simulink model "templateVFreplay"  (R2019b)
settings: Solver=ode23tb  StartTime=0  StopTime=dataSim(l).Time(end)  FixedStep=Ts
model workspace (MAT data in the model file):
  AC8B_test_sdosession : sldodialogs.data.SessionData (value not decoded)
  tp34291882_bceb_4da8_b486_81ba615ab517 = [0 0.0333333 0.0666667 0.1 0.1333334 0.1666667 0.2 0.2333333 0.2666666 0.2999999 0.3333332 0.3666665 ... (13500 elements, 2700x5)]
  tp5fd81924_c6b2_4820_a4c1_c746ac51258e : object (value not decoded)
  tp61e2f470_2812_498a_af75_e87b8b944307 = [0 0.0333333 0.0666667 0.1 0.1333334 0.1666667 0.2 0.2333333 0.2666666 0.2999999 0.3333332 0.3666665 ... (13500 elements, 2700x5)]
  tpfa3056f0_c430_45b3_969f_b76cef1498ad : object (value not decoded)
undefined symbols (not defined in the file): dataSim, dyn, Fnom, g, gcbh, genTpd0, genTppd0, genTppq0, genTpq0, genXd, genXl, genXpd, genXppd, genXppq, genXpq, genXq, govDisable, ifd, init, j, l, MBase, p, sps_rtmsupport, sys, Tb1, Tc1, Vnom, vt
libraries: powerlib x28, modelLibrary x22, simulink x15, powerlib_meascontrol x5, spsST2AModel x4, GenLib x2, ideal_source x1
(part 2 of 4)

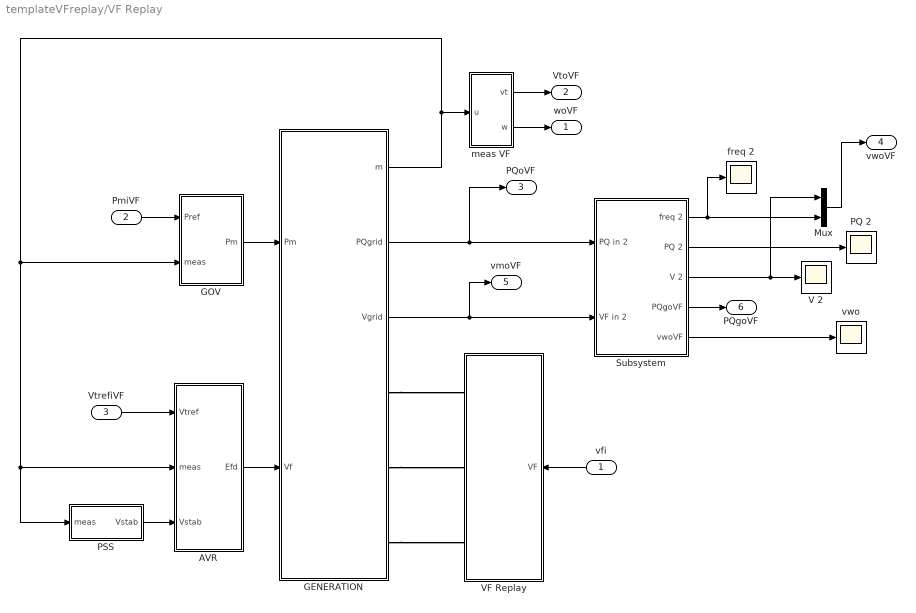
== system templateVFreplay/VF Replay ==
  vfi : Inport  PortDimensions=2
  PmiVF : Inport  Port=2
  VtrefiVF : Inport  Port=3
  AVR : Subsystem  BlockChoice=ST4B  VariantControlMode=Label  Variant=on  LabelModeActiveChoice=Variant1
      settings: AttributesFormatString=%<BlockChoice>
  GENERATION : Subsystem  VariantControlMode=Label  Variant=on  LabelModeActiveChoice=Variant2
      settings: AttributesFormatString=%<BlockChoice>
  GOV : Subsystem  BlockChoice=GGOV1  VariantControlMode=Label  Variant=on  LabelModeActiveChoice=Variant1
      settings: AttributesFormatString=%<BlockChoice>
  Mux : Mux  Inputs=2
  PQ 2 : Scope
  PSS : Subsystem  BlockChoice=PSS2B  VariantControlMode=Label  Variant=on  VariantControl=on  LabelModeActiveChoice=Variant2
      settings: AttributesFormatString=%<BlockChoice>
  Subsystem : Subsystem
  V 2 : Scope
  VF Replay : Subsystem
  freq 2 : Scope
  meas VF : Subsystem
  vwo : Scope
  woVF : Outport  VectorParamsAs1DForOutWhenUnconnected=off
  VtoVF : Outport  Port=2  VectorParamsAs1DForOutWhenUnconnected=off
  PQoVF : Outport  Port=3  SampleTime=1/30  VectorParamsAs1DForOutWhenUnconnected=off
  vwoVF : Outport  Port=4  VectorParamsAs1DForOutWhenUnconnected=off
  vmoVF : Outport  Port=5  VectorParamsAs1DForOutWhenUnconnected=off
  PQgoVF : Outport  Port=6  SampleTime=1/30  VectorParamsAs1DForOutWhenUnconnected=off
  wires:
  GENERATION/3(Vgrid) -> vmoVF/1, Subsystem/2(VF in 2)
  GENERATION/1(m) -> PSS/1(meas), AVR/2(meas), GOV/2(meas), meas VF/1(u)
  GENERATION/2(PQgrid) -> PQoVF/1, Subsystem/1(PQ in 2)
  vfi/1 -> VF Replay/1(VF)
  meas VF/1(vt) -> VtoVF/1
  meas VF/2(w) -> woVF/1
  Subsystem/1(freq 2) -> Mux/2, freq 2/1
  Subsystem/2(PQ 2) -> PQ 2/1
  Subsystem/4(PQgoVF) -> PQgoVF/1
  Subsystem/3(V 2) -> V 2/1, Mux/1
  Subsystem/5(vwoVF) -> vwo/1
  Mux/1 -> vwoVF/1
  VtrefiVF/1 -> AVR/1(Vtref)
  PmiVF/1 -> GOV/1(Pref)
  GOV/1(Pm) -> GENERATION/1(Pm)
  PSS/1(Vstab) -> AVR/3(Vstab)
  AVR/1(Efd) -> GENERATION/2(Vf)
  connections:
  GENERATION/RConn1 -- VF Replay/RConn1
  GENERATION/RConn2 -- VF Replay/RConn2
  GENERATION/RConn3 -- VF Replay/RConn3

== system templateVFreplay/view ==
  Gain : Gain  Gain=1/MBase
  Selector2 : Selector  InputPortWidth=4  IndexOptions=Index vector (dialog)  Indices=[2 4]  OutputSizes=1
  Selector3 : Selector  InputPortWidth=4  IndexOptions=Index vector (dialog)  Indices=[1 3]  OutputSizes=1
  P : Outport  VectorParamsAs1DForOutWhenUnconnected=off
  Q : Outport  Port=2  VectorParamsAs1DForOutWhenUnconnected=off
  wires:
  [PQ_2] -> Gain/1
  Gain/1 -> Selector2/1, Selector3/1
  Selector2/1 -> Q/1
  Selector3/1 -> P/1

== system templateVFreplay/VF Replay/AVR ==
  Vtref : Inport
  meas : Inport  Port=2
  Vstab : Inport  Port=3
  REXS : Subsystem  VariantControl=Variant1  mask{p=dyn.rexs_102_GAS}
      mask prompts: p "Parameters"
      mask DialogControl DescGroupVar Prompt: REXS
  ST1A : Subsystem  VariantControl=Variant2  mask{p=dyn.esst1a_102_HYDRO}
      mask prompts: p "Parameters"
      mask DialogControl DescGroupVar Prompt: ST1A
  ST4B : Subsystem  VariantControl=Variant3  mask{p=dyn.esst4b_102_STEAM}
      mask prompts: p "Parameters"
      mask DialogControl DescGroupVar Prompt: ST4B
  Efd : Outport  VectorParamsAs1DForOutWhenUnconnected=off

== system templateVFreplay/VF Replay/GENERATION ==
  Pm : Inport
  Vf : Inport  Port=2
  GENROU_TERMINAL : Subsystem  VariantControl=Variant1  mask{g=sys.GENERATOR(1), p=dyn.genrou_31923_COLUSGT1}
      mask prompts: g "Generator Parameters"; p "Dynamic Parameters"
      mask DialogControl DescGroupVar Prompt: GENROU_TRANSFORMER
  GENROU_TRANSFORMER : Subsystem  VariantControl=Variant2  mask{g=sys.GENERATOR(2), t=sys.TRANSFORMER, p=dyn.genrou_102_GAS}
      mask prompts: g "Generator Parameters"; t "Transformer Parameters"; p "Dynamic Parameters"
      mask DialogControl DescGroupVar Prompt: GENROU_TRANSFORMER
  GENSAL_TRANSFORMER : Subsystem  VariantControl=Variant3  mask{g=sys.GENERATOR(2), t=sys.TRANSFORMER, p=dyn.gentpj_102_HYDRO}
      mask prompts: g "Generator Parameters"; t "Transformer Parameters"; p "Dynamic Parameters"
      mask DialogControl DescGroupVar Prompt: GENSAL_TRANSFORMER
  GENTPJ_TERMINAL : Subsystem  VariantControl=Variant4  mask{g=g, t=t, p=p}
      mask prompts: g "Generator Parameters"; t "Transformer Parameters"; p "Dynamic Parameters"
      mask DialogControl DescGroupVar Prompt: GENTPJ_TRANSFORMER
  GENTPJ_TRANSFORMER : Subsystem  VariantControl=Variant5  mask{g=sys.GENERATOR(2), t=sys.TRANSFORMER, p=dyn.genrou_102_GAS}
      mask prompts: g "Generator Parameters"; t "Transformer Parameters"; p "Dynamic Parameters"
      mask DialogControl DescGroupVar Prompt: GENTPJ_TRANSFORMER
  A : PMIOPort  Side=Right
  B : PMIOPort  Port=2  Side=Right
  C : PMIOPort  Port=3  Side=Right
  m : Outport  VectorParamsAs1DForOutWhenUnconnected=off
  PQgrid : Outport  Port=2  VectorParamsAs1DForOutWhenUnconnected=off
  Vgrid : Outport  Port=3  VectorParamsAs1DForOutWhenUnconnected=off

== system templateVFreplay/VF Replay/GOV ==
  Pref : Inport
  meas : Inport  Port=2
  GGOV1 : Subsystem  VariantControl=Variant1  mask{p=dyn.ggov1_102_GAS, g=sys.GENERATOR(2)}
      mask prompts: p "Parameters"; g "generator"
      mask DialogControl DescGroupVar Prompt: GGOV1
  IEEEG3 : Subsystem  VariantControl=Variant2  mask{p=dyn.ieeeg3_102_HYDRO}
      mask prompts: p "Parameters"
      mask DialogControl DescGroupVar Prompt: IEEEG3
  Pm : Outport  VectorParamsAs1DForOutWhenUnconnected=off

== system templateVFreplay/VF Replay/PSS ==
  meas : Inport
  PSS1A : Subsystem  VariantControl=Variant1  mask{p=dyn.pss1a_102_HYDRO}
      mask prompts: p "Parameters"
      mask DialogControl DescGroupVar Prompt: PSS1A
  PSS2A : Subsystem  VariantControl=Variant2  mask{p=dyn.pss2a_102_GAS}
      mask prompts: p "Parameters"
      mask DialogControl DescGroupVar Prompt: PSS2A
  PSS2B : Subsystem  VariantControl=Variant3  mask{p=dyn.pss2b_102_STEAM}
      mask prompts: p "Parameters"
      mask DialogControl DescGroupVar Prompt: PSS2B
  Vstab : Outport  VectorParamsAs1DForOutWhenUnconnected=off

== system templateVFreplay/VF Replay/Subsystem ==
  PQ in 2 : Inport
  VF in 2 : Inport  Port=2
  PQ VF : Subsystem
  PQ VF comp : Subsystem
  V VF comp : Subsystem
  VF VF : Subsystem
  freq : Subsystem
  freq 2 : Outport  VectorParamsAs1DForOutWhenUnconnected=off
  PQ 2 : Outport  Port=2  VectorParamsAs1DForOutWhenUnconnected=off
  V 2 : Outport  Port=3  VectorParamsAs1DForOutWhenUnconnected=off
  PQgoVF : Outport  Port=4  VectorParamsAs1DForOutWhenUnconnected=off
  vwoVF : Outport  Port=5  VectorParamsAs1DForOutWhenUnconnected=off
  tag scope: PQ_2=global, PQoVF=global
  wires:
  V VF comp/1(y) -> V 2/1
  VF in 2/1 -> V VF comp/1(u), VF VF/1(u)
  PQ VF comp/1("y ") -> [PQ_2], PQ 2/1
  freq/1(y) -> freq 2/1
  PQ VF/1(y) -> PQgoVF/1
  VF VF/1(y) -> vwoVF/1
  PQ in 2/1 -> [PQoVF], PQ VF/1(u), PQ VF comp/1(u)

== system templateVFreplay/VF Replay/VF Replay ==
  VF : Inport
  Constant1 : Constant
  Demux : Demux  Outputs=2
  Gain : Gain  Gain=2*pi*60
  Gain7 : Gain  Gain=1e3*sqrt(2/3)
  Gain8 : Gain  Gain=2*pi*60
  Ideal Source (custom) : ideal_source/Ideal Source (custom)  InternalConnection=Yg  VoltagePhases=off  Voltage=sys.BUS(1).VBUS*1e3  PhaseAngle=0  Voltage_phases=[25e3 25e3 25e3]/sqrt(3)  PhaseAngles_phases=[0 -120 +120]  Frequency=60  NonIdealSource=on  SpecifyImpedance=off  Resistance=1e-5  Inductance=1e-5  ShortCircuitLevel=100e6  BaseVoltage=sys.BUS(1).VBUS*1e3  XRratio=7  BusType=swing  Pref=10e3  Qref=0  Prefabc=[10e3, 10e3, 10e3]  Qrefabc=[0, 0, 0]  Qmin=-inf  Qmax=inf
  Sum : Sum  Inputs=|+-
  theta integrator : Integrator  InitialCondition=2*pi*60
  theta integrator1 : Integrator  InitialCondition=2*pi*60
  A : PMIOPort  Side=Right
  B : PMIOPort  Port=2  Side=Right
  C : PMIOPort  Port=3  Side=Right
  wires:
  theta integrator/1 -> Sum/1
  Constant1/1 -> Gain8/1
  Gain7/1 -> Ideal Source (custom)/2
  VF/1 -> Demux/1
  Demux/2 -> Gain/1
  Gain/1 -> theta integrator/1
  Sum/1 -> Ideal Source (custom)/1
  Demux/1 -> Gain7/1
  theta integrator1/1 -> Sum/2
  Gain8/1 -> theta integrator1/1
  connections:
  Ideal Source (custom)/RConn2 -- B/RConn1
  Ideal Source (custom)/RConn1 -- C/RConn1
  Ideal Source (custom)/RConn3 -- A/RConn1

== system templateVFreplay/VF Replay/meas VF ==
  u : Inport
  Bus Selector6 : BusSelector  OutputSignals="dq0 components.Stator voltage  vd (pu),dq0 components.Stator voltage  vq (pu),Mechanical.Rotor speed  wm  (pu)"
  Euclidian Norm5 : Subsystem
  wo VF : Subsystem
  vt : Outport  VectorParamsAs1DForOutWhenUnconnected=off
  w : Outport  Port=2  VectorParamsAs1DForOutWhenUnconnected=off
  wires:
  u/1 -> Bus Selector6/1
  Bus Selector6/2 -> Euclidian Norm5/2(u2)  "<Stator voltage  vq (pu)>"
  Bus Selector6/1 -> Euclidian Norm5/1(u1)  "<Stator voltage  vd (pu)>"
  Euclidian Norm5/1(y) -> vt/1  "vt"
  Bus Selector6/3 -> wo VF/1(u)  "<Rotor speed  wm  (pu)>"
  wo VF/1(y) -> w/1

== system templateVFreplay/VF Replay/AVR/REXS ==
  Vtref : Inport
  meas : Inport  Port=2
  Vstab : Inport  Port=3
  Bus Selector1 : BusSelector  OutputSignals="dq0 components.Stator voltage  vd (pu),dq0 components.Stator voltage  vq (pu),dq0 components.Stator current  id (pu),dq0 components.Stator current  iq (pu),dq0 components.Field current  ifd (pu)"
  Euclidian Norm3 : Subsystem
  Euclidian Norm4 : Subsystem
  "Rotating Excitation System (Continuous) " : Subsystem  mask(PSS1A - Single Input Power System Stabilizer){Tr=p.tr, Kvp=p.kvp, Kvi=p.kvi, Vimax=p.vimax, Ta=p.ta, Tb=[p.tb1 p.tb2], Tc=[p.tc1 p.tc2], Vrrange=[p.vrmin p.vrmax], Kf=p.kf, Tf=p.tf, Tfll=[p.tf1 p.tf2], Fbf=p.fbf, Kip=p.kip, Kii=p.kii, Tp=p.tp, Kh=p.kh, Ke=p.ke, Te=p.te, Vfrange=[p.vfmin p.vfmax], Kc=p.kc, Kd=p.kd, E=[p.e1 p.e2], Se=[p.se1 p.se2], Xc=p.xc, Vcmax=p.vcmax, Kefd=p.kefd}
      mask prompts: Tr "Tr, Voltage Transducer Time Constant [s]"; Kvp "Kvp, Proportional Gain"; Kvi "Kvi, Integral Gain"; Vimax "Vimax, Input Limit [pu]"; Ta "Ta, Time Constant [s]"; Tb "Tb, Lag Time Constants [s]"; Tc "Tc, Lead Time Constants [s]"; Vrrange "[Vrmin Vrmax], Output Range [pu]"; Kf "Kf, Rate Gain"; Tf "Tf, Rate Time Constant [s]"; Tfll "[Tf1 Tf2], Lead/lag Contants [s]"; Fbf "Fbf, Feedback Signal Fl"; Kip "Kip, Regulator Proportional Gain"; Kii "Kii, Regulator Inegral Gain"; Tp "Tp, Bridge Time Constant [s]"; Kh "Kh, Voltage Controller Gain"; Ke "Ke, Exciter Proportional Constant"; Te "Te, Exciter Time Constant [s]"; Vfrange "[Vfmin Vfmax], Field Current Bounds [pu]"; Kc "Kc, Rectifier Regulation Factor [pu]"; Kd "Kd, Exciter Regulation Factor [pu]"; E "[E1 E2], Field Voltage Value Saturation"; Se "[Se1 Se2], Saturation Factor"; Xc "Xc,  Compounding Reactance [pu]"; Vcmax "Vcmax, Maximum Compounding Voltage [pu]"; Kefd "Kefd, Field Voltage Feedback"
      mask init:
      | % Extract Parameters
      | Tb1 = Tb(1);        Tb2 = Tb(2);
      | Tc1 = Tc(1);        Tc2 = Tc(2);
      | Tf1 = Tfll(1);      Tf2 = Tfll(2);
      | Vrmin = Vrrange(1); Vrmax = Vrrange(2);
      | Vfmin = Vfrange(1); Vfmax = Vfrange(2);
      mask DialogControl Container9 Prompt: Voltage Regulator
      mask DialogControl Container11 Prompt: Feedback Dynamics
      mask DialogControl Container25 Prompt: Field Current Regulator
      mask DialogControl Container29 Prompt: Rotating Exciter
      mask Display:
      | port_label('input',1,'Vref');
      | port_label('input',2,'Vt');
      | port_label('input',3,'It');
      | port_label('input',4,'Ifd');
      | port_label('input',5,'Vstab');
      | port_label('output',1,'Efd');
      | 
      | color('blue');disp('AVR/Exciter')
  Efd : Outport  VectorParamsAs1DForOutWhenUnconnected=off
  wires:
  Vstab/1 -> "Rotating Excitation System (Continuous) "/5(Vstab)
  Bus Selector1/1 -> Euclidian Norm3/1(u1)  "<Stator voltage  vd (pu)>"
  Vtref/1 -> "Rotating Excitation System (Continuous) "/1(Vref)
  Bus Selector1/3 -> Euclidian Norm4/1(u1)  "<Stator current  id (pu)>"
  Euclidian Norm4/1(y) -> "Rotating Excitation System (Continuous) "/3(It)  "It"
  Bus Selector1/4 -> Euclidian Norm4/2(u2)  "<Stator current  iq (pu)>"
  Bus Selector1/2 -> Euclidian Norm3/2(u2)  "<Stator voltage  vq (pu)>"
  Euclidian Norm3/1(y) -> "Rotating Excitation System (Continuous) "/2(Vt)  "Vt"
  Bus Selector1/5 -> "Rotating Excitation System (Continuous) "/4(Ifd)  "<Field current  ifd (pu)>"
  "Rotating Excitation System (Continuous) "/1(Efd) -> Efd/1
  meas/1 -> Bus Selector1/1

== system templateVFreplay/VF Replay/AVR/ST1A ==
  Vtref : Inport
  meas : Inport  Port=2
  Vstab : Inport  Port=3
  Bus Selector8 : BusSelector  OutputSignals="dq0 components.Field current  ifd (pu),dq0 components.Stator voltage  vd (pu),dq0 components.Stator voltage  vq (pu),dq0 components.Stator current  id (pu),dq0 components.Stator current  iq (pu)"
  Euclidian Norm1 : Subsystem
  Mux1 : Mux  Inputs=2
  Mux4 : Mux  Inputs=2
  ST1A Excitation System : Subsystem  DialogController=POWERSYS.PowerSysDialog  LoadFcn=sps_rtmsupport('LoadFcn', gcbh);  StartFcn=sps_rtmsupport('StartFcn', gcbh);  StopFcn=sps_rtmsupport('StopFcn', gcbh);  mask(ST1A Excitation System){Tr=20e-3, KaTa=[p.ka p.ta], VIminmax=[p.vimin p.vimax], VAminmax=[p.vamin p.vamax], VRminmax=[p.vrmin p.vrmax], KfTf=[p.kf p.tf], TbTc=[p.tb p.tc p.tb1 p.tc1], KLR=p.klr, ILR=p.ilr, Kc=p.kc, v0=[1 1], TsBlock=0}
      mask prompts: Tr "Low-pass filter time constant Tr(s):"; KaTa "Voltage regulator gain and time constant [Ka Ta(s)]:"; VIminmax "Voltage regulator input limits [VImin(pu) VImax(pu)]:"; VAminmax "Voltage regulator internal limits [VAmin(pu) VAmax(pu)]:"; VRminmax "Voltage regulator output limits [VRmin(pu) VRmax(pu)]:"; KfTf "Damping filter gain and time constant [Kf Tf(s)]:"; TbTc "Transient gain reduction lead and lag time constants [Tb(s) Tc(s) Tb1(s) Tc1(s)]:"; KLR "Exciter output current limiter gain KLR(pu):"; ILR "Exciter output current limit reference ILR(pu):"; Kc "Rectifier loading factor Kc(pu):"; v0 "Initial values of terminal voltage and field voltage [Vt0(pu) Efd0(pu)]:"; TsBlock "Sample time:"
      mask help: Implements a synchronous machine voltage regulator and exciter based on the IEEE type ST1A excitation system model. The output is the field voltage to apply to the Vf input of a Synchronous Machine block. Inputs and output are in p.u.
      mask init:
      | Ka = KaTa(1);
      | Ta = KaTa(2);
      | 
      | Kf = KfTf(1);
      | Tf = KfTf(2);
      | 
      | Tb = TbTc(1);
      | Tc = TbTc(2);
      settings: CopyFcn=sps_rtmsupport('CopyFcn', gcbh);  DeleteFcn=sps_rtmsupport('DeleteFcn', gcbh);  UndoDeleteFcn=sps_rtmsupport('UndoDeleteFcn', gcbh);  ModelCloseFcn=sps_rtmsupport('ModelCloseFcn', gcbh);  PreSaveFcn=sps_rtmsupport('PreSaveFcn', gcbh);  PostSaveFcn=sps_rtmsupport('PostSaveFcn', gcbh);  NameChangeFcn=sps_rtmsupport('NameChangeFcn', gcbh);  PreCopyFcn=sps_rtmsupport('PreCopyFcn', gcbh);  OpenFcn=sps_rtmsupport('OpenFcn', gcbh, []);  CloseFcn=sps_rtmsupport('CloseFcn', gcbh);  PreDeleteFcn=sps_rtmsupport('PreDeleteFcn', gcbh);
      mask Help: helpview(psbhelp);
      mask DialogControl ParameterTabVar0 Prompt: Controllers
      mask DialogControl ParameterTabVar01 Prompt: Exciter and Rectifier
      mask DialogControl ParameterTabVar012 Prompt: Initial Values
      mask Display: color('blue');disp('ST1A')
  Terminator : Terminator
  Efd : Outport  VectorParamsAs1DForOutWhenUnconnected=off
  wires:
  Mux1/1 -> Euclidian Norm1/1(u)
  Bus Selector8/3 -> Mux1/2  "<Stator voltage  vq (pu)>"
  Bus Selector8/2 -> Mux1/1  "<Stator voltage  vd (pu)>"
  Euclidian Norm1/1(y) -> ST1A Excitation System/2(Vt)
  meas/1 -> Bus Selector8/1
  Bus Selector8/4 -> Mux4/1  "<Stator current  id (pu)>"
  Bus Selector8/5 -> Mux4/2  "<Stator current  iq (pu)>"
  Vtref/1 -> ST1A Excitation System/1(Vref)
  Bus Selector8/1 -> ST1A Excitation System/3(Ifd)  "<Field current  ifd (pu)>"
  Vstab/1 -> ST1A Excitation System/4(Vstab)
  ST1A Excitation System/1(Efd) -> Efd/1
  Mux4/1 -> Terminator/1

== system templateVFreplay/VF Replay/AVR/ST4B ==
  Vtref : Inport
  meas : Inport  Port=2
  Vstab : Inport  Port=3
  Bus Selector8 : BusSelector  OutputSignals="dq0 components.Field current  ifd (pu),dq0 components.Stator voltage  vd (pu),dq0 components.Stator voltage  vq (pu),dq0 components.Stator current  id (pu),dq0 components.Stator current  iq (pu)"
  Euclidian Norm : Subsystem
  Euclidian Norm1 : Subsystem
  Mux1 : Mux  Inputs=2
  Mux4 : Mux  Inputs=2
  ST4B Excitation System (Continuous) : Subsystem  mask(ST4B Excitation System){Tr=p.tr, Kpr=p.kpr, Kir=p.kir, Ta=p.ta, Vrmax=p.vrmax, Vrmin=p.vrmin, Kpm=p.kpm, Kim=p.kim, Kg=p.kg, Vmmin=p.vmmin, Vmmax=p.vmmax, Vgmax=p.vgmax, Kp=p.kp, Ki=p.ki, Angp=p.angp, Kc=p.kc, Xl=p.xl, Vbmax=p.vbmax}
      mask prompts: Tr "Voltage Transducer Time (Tr)"; Kpr "AVR Proportional Gain (Kpr)"; Kir "AVR Integral Gain (Kir)"; Ta "AVR Time Constant (Ta) [sec]"; Vrmax "Maximum AVR Output (Vrmax)"; Vrmin "Minimum AVR Output (Vrmin)"; Kpm "Inner Loop Regulator P Gain (Kpm)"; Kim "Inner Loop Regulator I gain (Kim)"; Kg "Inner Loop Feedback Gain (Kg)"; Vmmin "Inner Loop Regulator Min Output (Vmmin)"; Vmmax "Inner Loop Regulator Max Output (Vmmax)"; Vgmax "Maximum inner loop feedback gain [Vgmax(pu)]"; Kp "Potential circuit gain coefficient (Kp)"; Ki "Current circuit gain coefficient (Ki)"; Angp "Potential Source Phase Angle [Angp (rad)]"; Kc "Rectifier loading factor (Kc)"; Xl "Leakage Reactance (XL)"; Vbmax "Maximum Excitation Voltage (Vbmax)"
      mask help:
      | Implements ST4B excitation system.
      |
      | Units of parameters are in PU unless otherwise noted.
      |
      | The ST4B Excitation System block currently only has a Continuous implementation and thus cannot have a specified sample time.
      mask DialogControl Container7 Prompt: Controllers
      mask DialogControl Container5 Prompt: Exciter and Rectifier
      mask Display: color('blue');disp('ST4B')
  Subsystem1 : Subsystem
  Subsystem2 : Subsystem
  Efd : Outport  VectorParamsAs1DForOutWhenUnconnected=off
  wires:
  ST4B Excitation System (Continuous)/1(Efd) -> Efd/1
  Bus Selector8/5 -> Mux4/2  "<Stator current  iq (pu)>"
  Bus Selector8/4 -> Mux4/1  "<Stator current  id (pu)>"
  Bus Selector8/1 -> ST4B Excitation System (Continuous)/2(Ifd)  "<Field current  ifd (pu)>"
  meas/1 -> Bus Selector8/1
  Vstab/1 -> ST4B Excitation System (Continuous)/4(Vs)
  Subsystem2/1(y) -> ST4B Excitation System (Continuous)/6(Vt_Ang)
  Euclidian Norm1/1(y) -> ST4B Excitation System (Continuous)/1(Vc), ST4B Excitation System (Continuous)/5(Vt)
  Subsystem1/1(y) -> ST4B Excitation System (Continuous)/8(It_Ang)
  Mux4/1 -> Euclidian Norm/1(u), Subsystem1/1(u)
  Euclidian Norm/1(y) -> ST4B Excitation System (Continuous)/7(It)
  Vtref/1 -> ST4B Excitation System (Continuous)/3(Vref)
  Bus Selector8/2 -> Mux1/1  "<Stator voltage  vd (pu)>"
  Bus Selector8/3 -> Mux1/2  "<Stator voltage  vq (pu)>"
  Mux1/1 -> Subsystem2/1(u), Euclidian Norm1/1(u)

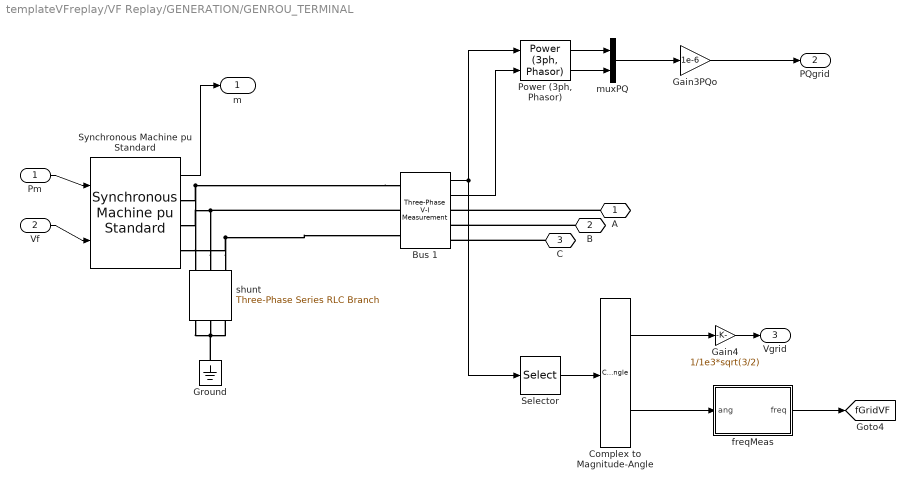
== system templateVFreplay/VF Replay/GENERATION/GENROU_TERMINAL ==
  Pm : Inport
  Vf : Inport  Port=2
  Bus 1 : powerlib/Measurements/Three-Phase V-I Measurement  VoltageMeasurement=phase-to-ground  SetLabelV=off  LabelV=Vabc  Vpu=off  VpuLL=off  CurrentMeasurement=yes  SetLabelI=off  LabelI=Iabc  Ipu=off  Pbase=100e6  Vbase=500e3  OutputType=Complex  PhasorSimulation=on  PSBequivalent=0
      settings: SourceProductName=Simscape Electrical
  Complex to Magnitude-Angle : ComplexToMagnitudeAngle
  Gain3PQo : Gain  Gain=1e-6
  Gain4 : Gain  Gain=1/1e3*sqrt(3/2)
  Ground : powerlib/Elements/Ground  LConnTagsString=a
      settings: SourceProductName=Simscape Electrical
  "Power (3ph, Phasor)" : powerlib_meascontrol/Measurements/Power (3ph, Phasor)
      settings: SourceProductName=Simscape Electrical  SourceProductBaseCode=PS
  Selector : Selector  InputPortWidth=3  IndexOptions=Index vector (dialog)  Indices=1  OutputSizes=1
  Synchronous Machine pu Standard : powerlib/Machines/Synchronous Machine pu Standard  PresetModel=No  MechanicalLoad=Mechanical power Pm  ShowDetailedParameters=on  RotorType=Round  Units=per unit standard parameters  MeasurementBus=off  NominalParameters=[g.MBASE*1e6 g.BUSV*1e3 60]  Reactances1=[p.ld p.lpd p.lppd p.lq p.lpq p.lppd p.ll-0.01]  Reactances2=[ genXd genXpd genXppd genXq genXpq genXppq genXl]  dAxisTimeConstants=Open-circuit  qAxisTimeConstants=Open-circuit  TimeConstants1="[ 4.4849  0.0681  0.1  ]"  TimeConstants2=[p.tpdo p.tppdo p.tpqo p.tppqo]  TimeConstants3="[  4.49  0.0681  0.0513  ]"  TimeConstants4=[ 8.0, 0.03, 0.3371, 0.0295 ]  TimeConstants5=[ 1.01, 0.053, 0.1 ]  TimeConstants6=[ 1.3201, 0.023, 1.0, 0.07 ]  TimeConstants7=[genTpd0 genTppd0 genTpq0 genTppq0]  TimeConstants8=[genTpd0 genTppd0 genTpq0 genTppq0]  StatorResistance=p.ra  Mechanical=[p.h p.d 2]  PolePairs=2  InitialConditions=[0 -89.4885 0.00587296 0.00587296 0.00587296 0 -120 120 1.00004]  SetSaturation=on  Saturation=[ifd; vt]  LoadFlowParameters=[2 0 0 0 0]  TsPowergui=0  TsBlock=-1  IterativeModel=Trapezoidal non iterative  IterativeDiscreteModel=Trapezoidal non iterative  BusType=PV  Pref=0  Qref=0  Qmin=-inf  Qmax=inf  PLF=0  QLF=0
      settings: SourceProductName=Simscape Electrical
  freqMeas : Subsystem
  muxPQ : Mux  Inputs=2
  shunt : powerlib/Elements/Three-Phase Series RLC Branch  LConnTagsString=A|B|C  RConnTagsString=A|B|C  BranchType=R  Resistance=1e6  Inductance=0.0025  Capacitance=0  Measurements=None
      settings: SourceProductName=Simscape Electrical
  A : PMIOPort  Side=Right
  B : PMIOPort  Port=2  Side=Right
  C : PMIOPort  Port=3  Side=Right
  m : Outport  VectorParamsAs1DForOutWhenUnconnected=off
  PQgrid : Outport  Port=2  VectorParamsAs1DForOutWhenUnconnected=off
  Vgrid : Outport  Port=3  VectorParamsAs1DForOutWhenUnconnected=off
  tag scope: fGridVF=global
  wires:
  muxPQ/1 -> Gain3PQo/1
  Bus 1/1 -> Selector/1, "Power (3ph, Phasor)"/1
  Bus 1/2 -> "Power (3ph, Phasor)"/2
  "Power (3ph, Phasor)"/1 -> muxPQ/1
  Pm/1 -> Synchronous Machine pu Standard/1
  Complex to Magnitude-Angle/1 -> Gain4/1
  Vf/1 -> Synchronous Machine pu Standard/2
  Gain3PQo/1 -> PQgrid/1
  Gain4/1 -> Vgrid/1
  "Power (3ph, Phasor)"/2 -> muxPQ/2
  Synchronous Machine pu Standard/1 -> m/1
  Selector/1 -> Complex to Magnitude-Angle/1
  Complex to Magnitude-Angle/2 -> freqMeas/1(ang)
  freqMeas/1(freq) -> [fGridVF]
  connections:
  shunt/LConn3 -- Bus 1/LConn3 -- Synchronous Machine pu Standard/RConn3
  Bus 1/LConn1 -- shunt/LConn1 -- Synchronous Machine pu Standard/RConn1
  shunt/LConn2 -- Bus 1/LConn2 -- Synchronous Machine pu Standard/RConn2
  A/RConn1 -- Bus 1/RConn1
  B/RConn1 -- Bus 1/RConn2
  C/RConn1 -- Bus 1/RConn3
  shunt/RConn1 -- Ground/LConn1 -- shunt/RConn2 -- shunt/RConn3

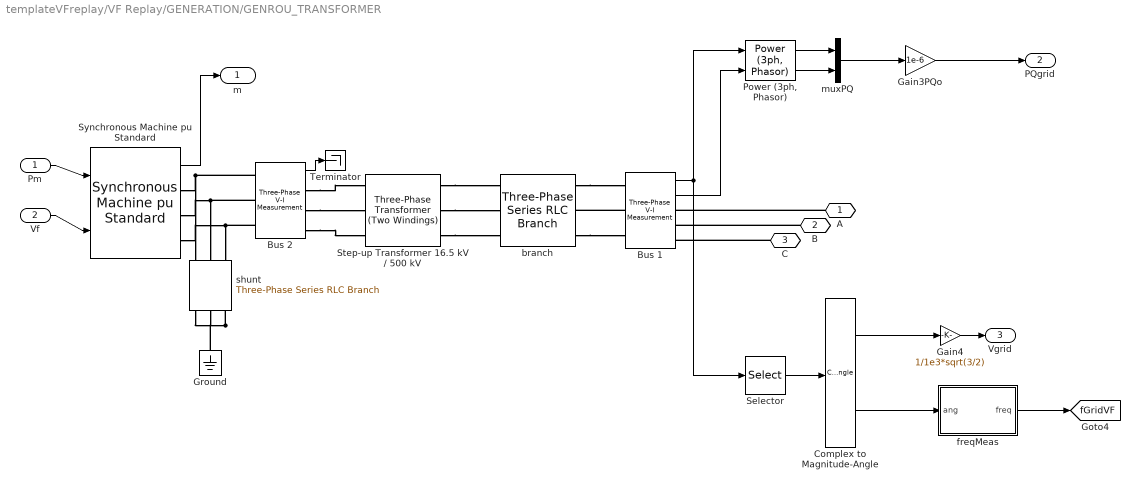
== system templateVFreplay/VF Replay/GENERATION/GENROU_TRANSFORMER ==
  Pm : Inport
  Vf : Inport  Port=2
  Bus 1 : powerlib/Measurements/Three-Phase V-I Measurement  VoltageMeasurement=phase-to-ground  SetLabelV=off  LabelV=Vabc  Vpu=off  VpuLL=off  CurrentMeasurement=yes  SetLabelI=off  LabelI=Iabc  Ipu=off  Pbase=100e6  Vbase=500e3  OutputType=Complex  PhasorSimulation=on  PSBequivalent=0
      settings: SourceProductName=Simscape Electrical
  Bus 2 : powerlib/Measurements/Three-Phase V-I Measurement  VoltageMeasurement=phase-to-ground  SetLabelV=off  LabelV=Vabc  Vpu=off  VpuLL=off  CurrentMeasurement=no  SetLabelI=off  LabelI=Iabc  Ipu=off  Pbase=100e6  Vbase=500e3  OutputType=Complex  PhasorSimulation=on  PSBequivalent=0
      settings: SourceProductName=Simscape Electrical
  Complex to Magnitude-Angle : ComplexToMagnitudeAngle
  Gain3PQo : Gain  Gain=1e-6
  Gain4 : Gain  Gain=1/1e3*sqrt(3/2)
  Ground : powerlib/Elements/Ground  LConnTagsString=a
      settings: SourceProductName=Simscape Electrical
  "Power (3ph, Phasor)" : powerlib_meascontrol/Measurements/Power (3ph, Phasor)
      settings: SourceProductName=Simscape Electrical  SourceProductBaseCode=PS
  Selector : Selector  InputPortWidth=3  IndexOptions=Index vector (dialog)  Indices=1  OutputSizes=1
  Step-up Transformer 16.5 kV / 500 kV : powerlib/Elements/Three-Phase Transformer (Two Windings)  Winding1Connection=Yg  Winding2Connection=Yg  CoreType=Three single-phase transformers  SetSaturation=off  Hysteresis=off  DataFile='hysteresis'  SetInitialFlux=off  Measurements=None  UNITS=pu  NominalPower=[t.TBASE*1e6 60 ]  Winding1="[t.JV*1e3 t.PS_R/2  t.PS_X/2]"  Winding2="[t.IV*1e3 t.PS_R/2  t.PS_X/2]"  Rm=1/t.GMAG  Lm=1/abs(t.BMAG)  L0=0.5  Saturation="[ 0,0  ;  0.005,1.2  ;  1.0,1.4 ]"  InitialFluxes=[ 0.8 , -0.8 , 0.7 ]  BreakLoop=off  DiscreteSolver=Trapezoidal iterative  DataType=off  TransfoNumber=0
      settings: SourceProductName=Simscape Electrical
  Synchronous Machine pu Standard : powerlib/Machines/Synchronous Machine pu Standard  PresetModel=No  MechanicalLoad=Mechanical power Pm  ShowDetailedParameters=on  RotorType=Round  Units=per unit standard parameters  MeasurementBus=off  NominalParameters=[g.MBASE*1e6 g.BUSV*1e3 60]  Reactances1=[p.ld p.lpd p.lppd p.lq p.lpq p.lppd p.ll-0.01]  Reactances2=[ genXd genXpd genXppd genXq genXpq genXppq genXl]  dAxisTimeConstants=Open-circuit  qAxisTimeConstants=Open-circuit  TimeConstants1="[ 4.4849  0.0681  0.1  ]"  TimeConstants2=[p.tpdo p.tppdo p.tpqo p.tppqo]  TimeConstants3="[  4.49  0.0681  0.0513  ]"  TimeConstants4=[ 8.0, 0.03, 0.3371, 0.0295 ]  TimeConstants5=[ 1.01, 0.053, 0.1 ]  TimeConstants6=[ 1.3201, 0.023, 1.0, 0.07 ]  TimeConstants7=[genTpd0 genTppd0 genTpq0 genTppq0]  TimeConstants8=[genTpd0 genTppd0 genTpq0 genTppq0]  StatorResistance=p.ra  Mechanical=[p.h p.d 2]  PolePairs=2  InitialConditions=[0 -89.4885 0.00587296 0.00587296 0.00587296 0 -120 120 1.00004]  SetSaturation=on  Saturation=[ifd; vt]  LoadFlowParameters=[2 0 0 0 0]  TsPowergui=0  TsBlock=-1  IterativeModel=Trapezoidal non iterative  IterativeDiscreteModel=Trapezoidal non iterative  BusType=PV  Pref=0  Qref=0  Qmin=-inf  Qmax=inf  PLF=0  QLF=0
      settings: SourceProductName=Simscape Electrical
  Terminator : Terminator
  branch : powerlib/Elements/Three-Phase Series RLC Branch  LConnTagsString=A|B|C  RConnTagsString=A|B|C  BranchType=L  Resistance=0  Inductance=0.0003*500e3^2/100e6/2/pi/60  Capacitance=0  Measurements=None
      settings: SourceProductName=Simscape Electrical
  freqMeas : Subsystem
  muxPQ : Mux  Inputs=2
  shunt : powerlib/Elements/Three-Phase Series RLC Branch  LConnTagsString=A|B|C  RConnTagsString=A|B|C  BranchType=R  Resistance=1e6  Inductance=0.0025  Capacitance=0  Measurements=None
      settings: SourceProductName=Simscape Electrical
  A : PMIOPort  Side=Right
  B : PMIOPort  Port=2  Side=Right
  C : PMIOPort  Port=3  Side=Right
  m : Outport  VectorParamsAs1DForOutWhenUnconnected=off
  PQgrid : Outport  Port=2  VectorParamsAs1DForOutWhenUnconnected=off
  Vgrid : Outport  Port=3  VectorParamsAs1DForOutWhenUnconnected=off
  tag scope: fGridVF=global
  wires:
  freqMeas/1(freq) -> [fGridVF]
  Complex to Magnitude-Angle/2 -> freqMeas/1(ang)
  Selector/1 -> Complex to Magnitude-Angle/1
  Synchronous Machine pu Standard/1 -> m/1
  "Power (3ph, Phasor)"/2 -> muxPQ/2
  Gain4/1 -> Vgrid/1
  Gain3PQo/1 -> PQgrid/1
  Vf/1 -> Synchronous Machine pu Standard/2
  Complex to Magnitude-Angle/1 -> Gain4/1
  Pm/1 -> Synchronous Machine pu Standard/1
  "Power (3ph, Phasor)"/1 -> muxPQ/1
  Bus 1/2 -> "Power (3ph, Phasor)"/2
  Bus 1/1 -> "Power (3ph, Phasor)"/1, Selector/1
  muxPQ/1 -> Gain3PQo/1
  Bus 2/1 -> Terminator/1
  connections:
  Step-up Transformer 16.5 kV / 500 kV/RConn3 -- branch/LConn3
  Bus 1/LConn2 -- branch/RConn2
  shunt/RConn3 -- shunt/RConn2 -- Ground/LConn1 -- shunt/RConn1
  Step-up Transformer 16.5 kV / 500 kV/RConn2 -- branch/LConn2
  C/RConn1 -- Bus 1/RConn3
  branch/RConn1 -- Bus 1/LConn1
  branch/RConn3 -- Bus 1/LConn3
  B/RConn1 -- Bus 1/RConn2
  A/RConn1 -- Bus 1/RConn1
  Step-up Transformer 16.5 kV / 500 kV/RConn1 -- branch/LConn1
  Synchronous Machine pu Standard/RConn1 -- Bus 2/LConn1 -- shunt/LConn1
  Synchronous Machine pu Standard/RConn2 -- Bus 2/LConn2 -- shunt/LConn2
  Synchronous Machine pu Standard/RConn3 -- Bus 2/LConn3 -- shunt/LConn3
  Bus 2/RConn1 -- Step-up Transformer 16.5 kV / 500 kV/LConn1
  Bus 2/RConn2 -- Step-up Transformer 16.5 kV / 500 kV/LConn2
  Bus 2/RConn3 -- Step-up Transformer 16.5 kV / 500 kV/LConn3

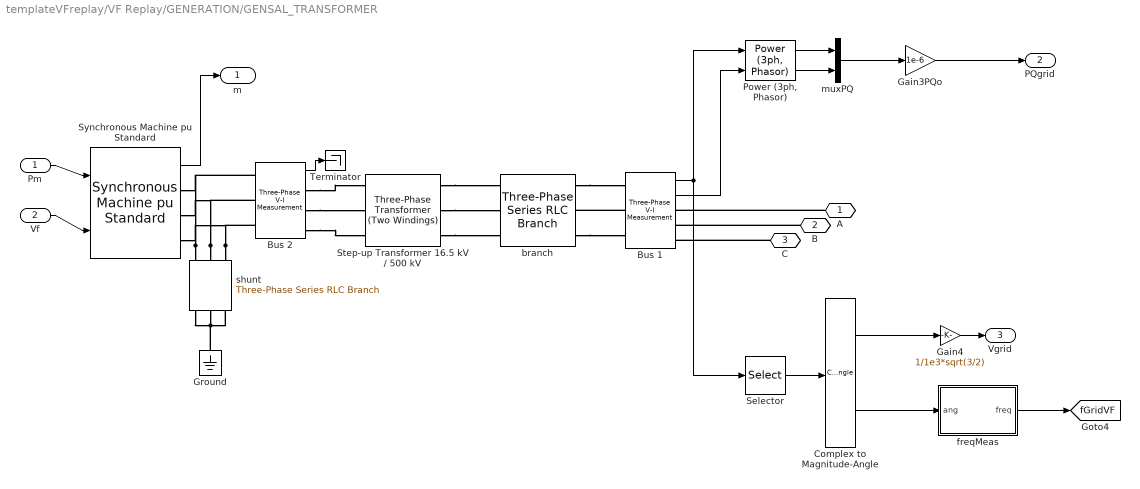
== system templateVFreplay/VF Replay/GENERATION/GENSAL_TRANSFORMER ==
  Pm : Inport
  Vf : Inport  Port=2
  Bus 1 : powerlib/Measurements/Three-Phase V-I Measurement  VoltageMeasurement=phase-to-ground  SetLabelV=off  LabelV=Vabc  Vpu=off  VpuLL=off  CurrentMeasurement=yes  SetLabelI=off  LabelI=Iabc  Ipu=off  Pbase=100e6  Vbase=500e3  OutputType=Complex  PhasorSimulation=on  PSBequivalent=0
      settings: SourceProductName=Simscape Electrical
  Bus 2 : powerlib/Measurements/Three-Phase V-I Measurement  VoltageMeasurement=phase-to-ground  SetLabelV=off  LabelV=Vabc  Vpu=off  VpuLL=off  CurrentMeasurement=no  SetLabelI=off  LabelI=Iabc  Ipu=off  Pbase=100e6  Vbase=500e3  OutputType=Complex  PhasorSimulation=on  PSBequivalent=0
      settings: SourceProductName=Simscape Electrical
  Complex to Magnitude-Angle : ComplexToMagnitudeAngle
  Gain3PQo : Gain  Gain=1e-6
  Gain4 : Gain  Gain=1/1e3*sqrt(3/2)
  Ground : powerlib/Elements/Ground  LConnTagsString=a
      settings: SourceProductName=Simscape Electrical
  "Power (3ph, Phasor)" : powerlib_meascontrol/Measurements/Power (3ph, Phasor)
      settings: SourceProductName=Simscape Electrical  SourceProductBaseCode=PS
  Selector : Selector  InputPortWidth=3  IndexOptions=Index vector (dialog)  Indices=1  OutputSizes=1
  Step-up Transformer 16.5 kV / 500 kV : powerlib/Elements/Three-Phase Transformer (Two Windings)  Winding1Connection=Yg  Winding2Connection=Yg  CoreType=Three single-phase transformers  SetSaturation=off  Hysteresis=off  DataFile='hysteresis'  SetInitialFlux=off  Measurements=None  UNITS=pu  NominalPower=[t.TBASE*1e6 60 ]  Winding1="[t.JV*1e3 t.PS_R/2  t.PS_X/2]"  Winding2="[t.IV*1e3 t.PS_R/2  t.PS_X/2]"  Rm=1/t.GMAG  Lm=1/abs(t.BMAG)  L0=0.5  Saturation="[ 0,0  ;  0.005,1.2  ;  1.0,1.4 ]"  InitialFluxes=[ 0.8 , -0.8 , 0.7 ]  BreakLoop=off  DiscreteSolver=Trapezoidal iterative  DataType=off  TransfoNumber=0
      settings: SourceProductName=Simscape Electrical
  Synchronous Machine pu Standard : powerlib/Machines/Synchronous Machine pu Standard  PresetModel=No  MechanicalLoad=Mechanical power Pm  ShowDetailedParameters=on  RotorType=Salient-pole  Units=per unit standard parameters  MeasurementBus=off  NominalParameters=[g.MBASE*1e6 g.BUSV*1e3 60]  Reactances1=[p.ld p.lpd p.lppd p.lq p.lpq p.lppd p.ll-0.01]  Reactances2=[p.ld p.lpd p.lppd p.lq p.lppq p.ll]  dAxisTimeConstants=Open-circuit  qAxisTimeConstants=Open-circuit  TimeConstants1=[p.tpdo p.tppdo p.tppqo]  TimeConstants2=[p.tpdo p.tppdo p.tpqo p.tppqo]  TimeConstants3="[  4.49  0.0681  0.0513  ]"  TimeConstants4=[ 8.0, 0.03, 0.3371, 0.0295 ]  TimeConstants5=[ 1.01, 0.053, 0.1 ]  TimeConstants6=[ 1.3201, 0.023, 1.0, 0.07 ]  TimeConstants7=[genTpd0 genTppd0 genTpq0 genTppq0]  TimeConstants8=[genTpd0 genTppd0 genTpq0 genTppq0]  StatorResistance=p.ra  Mechanical=[p.h p.d 2]  PolePairs=2  InitialConditions=[0 -89.4885 0.00587296 0.00587296 0.00587296 0 -120 120 1.00004]  SetSaturation=on  Saturation=[ifd; vt]  LoadFlowParameters=[2 0 0 0 0]  TsPowergui=0  TsBlock=-1  IterativeModel=Trapezoidal non iterative  IterativeDiscreteModel=Trapezoidal non iterative  BusType=PV  Pref=0  Qref=0  Qmin=-inf  Qmax=inf  PLF=0  QLF=0
      settings: SourceProductName=Simscape Electrical
  Terminator : Terminator
  branch : powerlib/Elements/Three-Phase Series RLC Branch  LConnTagsString=A|B|C  RConnTagsString=A|B|C  BranchType=L  Resistance=0  Inductance=0.0003*500e3^2/100e6/2/pi/60  Capacitance=0  Measurements=None
      settings: SourceProductName=Simscape Electrical
  freqMeas : Subsystem
  muxPQ : Mux  Inputs=2
  shunt : powerlib/Elements/Three-Phase Series RLC Branch  LConnTagsString=A|B|C  RConnTagsString=A|B|C  BranchType=R  Resistance=1e6  Inductance=0.0025  Capacitance=0  Measurements=None
      settings: SourceProductName=Simscape Electrical
  A : PMIOPort  Side=Right
  B : PMIOPort  Port=2  Side=Right
  C : PMIOPort  Port=3  Side=Right
  m : Outport  VectorParamsAs1DForOutWhenUnconnected=off
  PQgrid : Outport  Port=2  VectorParamsAs1DForOutWhenUnconnected=off
  Vgrid : Outport  Port=3  VectorParamsAs1DForOutWhenUnconnected=off
  tag scope: fGridVF=global
  wires:
  Bus 2/1 -> Terminator/1
  muxPQ/1 -> Gain3PQo/1
  Bus 1/1 -> Selector/1, "Power (3ph, Phasor)"/1
  Bus 1/2 -> "Power (3ph, Phasor)"/2
  "Power (3ph, Phasor)"/1 -> muxPQ/1
  Pm/1 -> Synchronous Machine pu Standard/1
  Complex to Magnitude-Angle/1 -> Gain4/1
  Vf/1 -> Synchronous Machine pu Standard/2
  Gain3PQo/1 -> PQgrid/1
  Gain4/1 -> Vgrid/1
  "Power (3ph, Phasor)"/2 -> muxPQ/2
  Synchronous Machine pu Standard/1 -> m/1
  Selector/1 -> Complex to Magnitude-Angle/1
  Complex to Magnitude-Angle/2 -> freqMeas/1(ang)
  freqMeas/1(freq) -> [fGridVF]
  connections:
  Bus 2/RConn3 -- Step-up Transformer 16.5 kV / 500 kV/LConn3
  Bus 2/RConn2 -- Step-up Transformer 16.5 kV / 500 kV/LConn2
  Bus 2/RConn1 -- Step-up Transformer 16.5 kV / 500 kV/LConn1
  shunt/LConn3 -- Bus 2/LConn3 -- Synchronous Machine pu Standard/RConn3
  shunt/LConn2 -- Bus 2/LConn2 -- Synchronous Machine pu Standard/RConn2
  shunt/LConn1 -- Bus 2/LConn1 -- Synchronous Machine pu Standard/RConn1
  Step-up Transformer 16.5 kV / 500 kV/RConn1 -- branch/LConn1
  A/RConn1 -- Bus 1/RConn1
  B/RConn1 -- Bus 1/RConn2
  branch/RConn3 -- Bus 1/LConn3
  branch/RConn1 -- Bus 1/LConn1
  C/RConn1 -- Bus 1/RConn3
  Step-up Transformer 16.5 kV / 500 kV/RConn2 -- branch/LConn2
  shunt/RConn1 -- Ground/LConn1 -- shunt/RConn2 -- shunt/RConn3
  Bus 1/LConn2 -- branch/RConn2
  Step-up Transformer 16.5 kV / 500 kV/RConn3 -- branch/LConn3

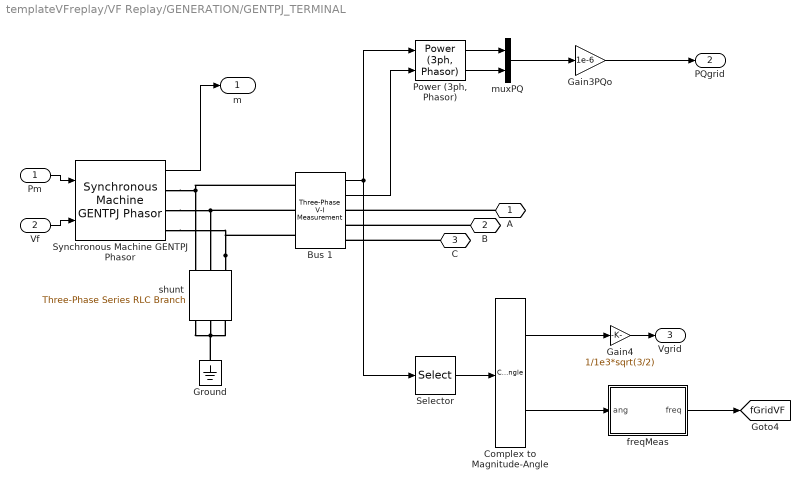
== system templateVFreplay/VF Replay/GENERATION/GENTPJ_TERMINAL ==
  Pm : Inport
  Vf : Inport  Port=2
  Bus 1 : powerlib/Measurements/Three-Phase V-I Measurement  VoltageMeasurement=phase-to-ground  SetLabelV=off  LabelV=Vabc  Vpu=off  VpuLL=off  CurrentMeasurement=yes  SetLabelI=off  LabelI=Iabc  Ipu=off  Pbase=100e6  Vbase=500e3  OutputType=Complex  PhasorSimulation=on  PSBequivalent=0
      settings: SourceProductName=Simscape Electrical
  Complex to Magnitude-Angle : ComplexToMagnitudeAngle
  Gain3PQo : Gain  Gain=1e-6
  Gain4 : Gain  Gain=1/1e3*sqrt(3/2)
  Ground : powerlib/Elements/Ground  LConnTagsString=a
      settings: SourceProductName=Simscape Electrical
  "Power (3ph, Phasor)" : powerlib_meascontrol/Measurements/Power (3ph, Phasor)
      settings: SourceProductName=Simscape Electrical  SourceProductBaseCode=PS
  Selector : Selector  InputPortWidth=3  IndexOptions=Index vector (dialog)  Indices=1  OutputSizes=1
  Synchronous Machine GENTPJ Phasor : GenLib/Synchronous Machine GENTPJ Phasor  PresetModel=No  MechanicalLoad=Mechanical power Pm  ShowDetailedParameters=on  RotorType=Salient-pole  Units=per unit fundamental parameters  MeasurementBus=off  NominalParameters="[ 187E6  13800   60]"  Stator="[ 2.85E-03  0.114  1.19  0.36 ]"  Field="[ 5.79E-04  0.114]"  Dampers2=[0.0652, 0.5134, 0.0287, 0.2553, 7.765e-3, 0.9167 ]  Dampers1="[ 1.17E-02  0.182  1.97E-02  0.384 ]"  Mechanical=[ 3.7 0 20]  PolePairs=20  InitialConditions="[ 0  0  0  0  0  0  0  0  1 ]"  SetSaturation=off  Saturation=[0.6404,0.7127,0.8441,0.9214,0.9956,1.082,1.19,1.316,1.457;0.7,0.7698,0.8872,0.9466,0.9969,1.046,1.1,1.151,1.201]  LoadFlowParameters=[1,0,0,0,0]  TsPowergui=0  TsBlock=-1  IterativeModel=Trapezoidal non iterative  IterativeDiscreteModel=Trapezoidal non iterative  BusType=PV  Pref=0  Qref=0  Qmin=-inf  Qmax=inf  PLF=0  QLF=0  Pnom=g.MBASE*1e6  Vnom=g.BUSV*1e3  fnom=60  Ra=p.ra  Xl=p.ll  Xd=p.ld  Xq=p.lq  Xdp=p.lpd  Xqp=p.lpq  Xdpp=p.lppd  Xqpp=p.lppq  Tdop=p.tpdo  Tqop=p.tpqo  Tdopp=p.tppdo  Tqopp=p.tppqo  SatOption=Quadratic  Ifd=[0 0.5 0.6 0.7 0.8 0.9 1 1.0562 1.1184 1.1985 1.2994 1.4576 1.6524 2.2234]  Vag=[0 0.5 0.6 0.7 0.8 0.9 0.995 1.05 1.1 1.15 1.2 1.25 1.3 1.4]  S10S12=[p.s1 p.s12]  Kis=p.kis  SatOn=on  InputType=Mechanical power Pm  H=p.h  D=p.d
  freqMeas : Subsystem
  muxPQ : Mux  Inputs=2
  shunt : powerlib/Elements/Three-Phase Series RLC Branch  LConnTagsString=A|B|C  RConnTagsString=A|B|C  BranchType=R  Resistance=1e6  Inductance=0.0025  Capacitance=0  Measurements=None
      settings: SourceProductName=Simscape Electrical
  A : PMIOPort  Side=Right
  B : PMIOPort  Port=2  Side=Right
  C : PMIOPort  Port=3  Side=Right
  m : Outport  VectorParamsAs1DForOutWhenUnconnected=off
  PQgrid : Outport  Port=2  VectorParamsAs1DForOutWhenUnconnected=off
  Vgrid : Outport  Port=3  VectorParamsAs1DForOutWhenUnconnected=off
  tag scope: fGridVF=global
  wires:
  muxPQ/1 -> Gain3PQo/1
  Bus 1/1 -> Selector/1, "Power (3ph, Phasor)"/1
  Bus 1/2 -> "Power (3ph, Phasor)"/2
  "Power (3ph, Phasor)"/1 -> muxPQ/1
  Pm/1 -> Synchronous Machine GENTPJ Phasor/1
  Complex to Magnitude-Angle/1 -> Gain4/1
  Vf/1 -> Synchronous Machine GENTPJ Phasor/2
  Gain3PQo/1 -> PQgrid/1
  Gain4/1 -> Vgrid/1
  "Power (3ph, Phasor)"/2 -> muxPQ/2
  Synchronous Machine GENTPJ Phasor/1 -> m/1
  Selector/1 -> Complex to Magnitude-Angle/1
  Complex to Magnitude-Angle/2 -> freqMeas/1(ang)
  freqMeas/1(freq) -> [fGridVF]
  connections:
  shunt/LConn3 -- Bus 1/LConn3 -- Synchronous Machine GENTPJ Phasor/RConn3
  Bus 1/LConn2 -- shunt/LConn2 -- Synchronous Machine GENTPJ Phasor/RConn2
  Bus 1/LConn1 -- shunt/LConn1 -- Synchronous Machine GENTPJ Phasor/RConn1
  A/RConn1 -- Bus 1/RConn1
  B/RConn1 -- Bus 1/RConn2
  C/RConn1 -- Bus 1/RConn3
  shunt/RConn1 -- Ground/LConn1 -- shunt/RConn2 -- shunt/RConn3

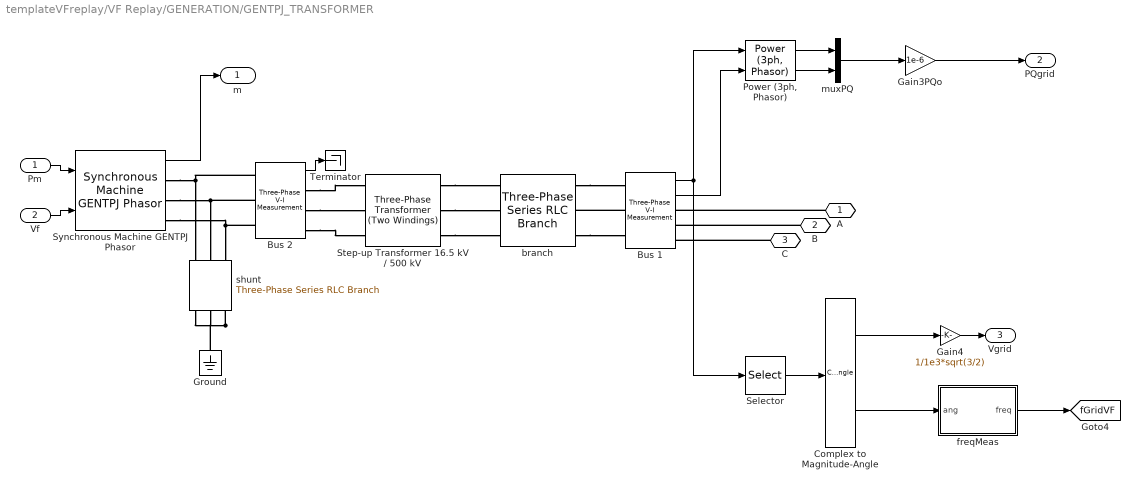
== system templateVFreplay/VF Replay/GENERATION/GENTPJ_TRANSFORMER ==
  Pm : Inport
  Vf : Inport  Port=2
  Bus 1 : powerlib/Measurements/Three-Phase V-I Measurement  VoltageMeasurement=phase-to-ground  SetLabelV=off  LabelV=Vabc  Vpu=off  VpuLL=off  CurrentMeasurement=yes  SetLabelI=off  LabelI=Iabc  Ipu=off  Pbase=100e6  Vbase=500e3  OutputType=Complex  PhasorSimulation=on  PSBequivalent=0
      settings: SourceProductName=Simscape Electrical
  Bus 2 : powerlib/Measurements/Three-Phase V-I Measurement  VoltageMeasurement=phase-to-ground  SetLabelV=off  LabelV=Vabc  Vpu=off  VpuLL=off  CurrentMeasurement=no  SetLabelI=off  LabelI=Iabc  Ipu=off  Pbase=100e6  Vbase=500e3  OutputType=Complex  PhasorSimulation=on  PSBequivalent=0
      settings: SourceProductName=Simscape Electrical
  Complex to Magnitude-Angle : ComplexToMagnitudeAngle
  Gain3PQo : Gain  Gain=1e-6
  Gain4 : Gain  Gain=1/1e3*sqrt(3/2)
  Ground : powerlib/Elements/Ground  LConnTagsString=a
      settings: SourceProductName=Simscape Electrical
  "Power (3ph, Phasor)" : powerlib_meascontrol/Measurements/Power (3ph, Phasor)
      settings: SourceProductName=Simscape Electrical  SourceProductBaseCode=PS
  Selector : Selector  InputPortWidth=3  IndexOptions=Index vector (dialog)  Indices=1  OutputSizes=1
  Step-up Transformer 16.5 kV / 500 kV : powerlib/Elements/Three-Phase Transformer (Two Windings)  Winding1Connection=Yg  Winding2Connection=Yg  CoreType=Three single-phase transformers  SetSaturation=off  Hysteresis=off  DataFile='hysteresis'  SetInitialFlux=off  Measurements=None  UNITS=pu  NominalPower=[t.TBASE*1e6 60 ]  Winding1="[t.JV*1e3 t.PS_R/2  t.PS_X/2]"  Winding2="[t.IV*1e3 t.PS_R/2  t.PS_X/2]"  Rm=1/t.GMAG  Lm=1/abs(t.BMAG)  L0=0.5  Saturation="[ 0,0  ;  0.005,1.2  ;  1.0,1.4 ]"  InitialFluxes=[ 0.8 , -0.8 , 0.7 ]  BreakLoop=off  DiscreteSolver=Trapezoidal iterative  DataType=off  TransfoNumber=0
      settings: SourceProductName=Simscape Electrical
  Synchronous Machine GENTPJ Phasor : GenLib/Synchronous Machine GENTPJ Phasor  PresetModel=No  MechanicalLoad=Mechanical power Pm  ShowDetailedParameters=on  RotorType=Salient-pole  Units=per unit fundamental parameters  MeasurementBus=off  NominalParameters="[ 187E6  13800   60]"  Stator="[ 2.85E-03  0.114  1.19  0.36 ]"  Field="[ 5.79E-04  0.114]"  Dampers2=[0.0652, 0.5134, 0.0287, 0.2553, 7.765e-3, 0.9167 ]  Dampers1="[ 1.17E-02  0.182  1.97E-02  0.384 ]"  Mechanical=[ 3.7 0 20]  PolePairs=20  InitialConditions="[ 0  0  0  0  0  0  0  0  1 ]"  SetSaturation=on  Saturation=[0.6404,0.7127,0.8441,0.9214,0.9956,1.082,1.19,1.316,1.457;0.7,0.7698,0.8872,0.9466,0.9969,1.046,1.1,1.151,1.201]  LoadFlowParameters=[1,0,0,0,0]  TsPowergui=0  TsBlock=-1  IterativeModel=Trapezoidal non iterative  IterativeDiscreteModel=Trapezoidal non iterative  BusType=PV  Pref=0  Qref=0  Qmin=-inf  Qmax=inf  PLF=0  QLF=0  Pnom=g.MBASE*1e6  Vnom=g.BUSV*1e3  fnom=60  Ra=p.ra  Xl=p.ll  Xd=p.ld  Xq=p.lq  Xdp=p.lpd  Xqp=p.lpq  Xdpp=p.lppd  Xqpp=p.lppq  Tdop=p.tpdo  Tqop=p.tpqo  Tdopp=p.tppdo  Tqopp=p.tppqo  SatOption=Quadratic  Ifd=[0 0.5 0.6 0.7 0.8 0.9 1 1.0562 1.1184 1.1985 1.2994 1.4576 1.6524 2.2234]  Vag=[0 0.5 0.6 0.7 0.8 0.9 0.995 1.05 1.1 1.15 1.2 1.25 1.3 1.4]  S10S12=[p.s1 p.s12]  Kis=p.kis  SatOn=on  InputType=Mechanical power Pm  H=p.h  D=p.d
  Terminator : Terminator
  branch : powerlib/Elements/Three-Phase Series RLC Branch  LConnTagsString=A|B|C  RConnTagsString=A|B|C  BranchType=L  Resistance=0  Inductance=0.0003*500e3^2/100e6/2/pi/60  Capacitance=0  Measurements=None
      settings: SourceProductName=Simscape Electrical
  freqMeas : Subsystem
  muxPQ : Mux  Inputs=2
  shunt : powerlib/Elements/Three-Phase Series RLC Branch  LConnTagsString=A|B|C  RConnTagsString=A|B|C  BranchType=R  Resistance=1e6  Inductance=0.0025  Capacitance=0  Measurements=None
      settings: SourceProductName=Simscape Electrical
  A : PMIOPort  Side=Right
  B : PMIOPort  Port=2  Side=Right
  C : PMIOPort  Port=3  Side=Right
  m : Outport  VectorParamsAs1DForOutWhenUnconnected=off
  PQgrid : Outport  Port=2  VectorParamsAs1DForOutWhenUnconnected=off
  Vgrid : Outport  Port=3  VectorParamsAs1DForOutWhenUnconnected=off
  tag scope: fGridVF=global
  wires:
  freqMeas/1(freq) -> [fGridVF]
  Complex to Magnitude-Angle/2 -> freqMeas/1(ang)
  Selector/1 -> Complex to Magnitude-Angle/1
  Synchronous Machine GENTPJ Phasor/1 -> m/1
  "Power (3ph, Phasor)"/2 -> muxPQ/2
  Gain4/1 -> Vgrid/1
  Gain3PQo/1 -> PQgrid/1
  Vf/1 -> Synchronous Machine GENTPJ Phasor/2
  Complex to Magnitude-Angle/1 -> Gain4/1
  Pm/1 -> Synchronous Machine GENTPJ Phasor/1
  "Power (3ph, Phasor)"/1 -> muxPQ/1
  Bus 1/2 -> "Power (3ph, Phasor)"/2
  Bus 1/1 -> "Power (3ph, Phasor)"/1, Selector/1
  muxPQ/1 -> Gain3PQo/1
  Bus 2/1 -> Terminator/1
  connections:
  Step-up Transformer 16.5 kV / 500 kV/RConn3 -- branch/LConn3
  Bus 1/LConn2 -- branch/RConn2
  shunt/RConn3 -- shunt/RConn2 -- Ground/LConn1 -- shunt/RConn1
  Step-up Transformer 16.5 kV / 500 kV/RConn2 -- branch/LConn2
  C/RConn1 -- Bus 1/RConn3
  branch/RConn1 -- Bus 1/LConn1
  branch/RConn3 -- Bus 1/LConn3
  B/RConn1 -- Bus 1/RConn2
  A/RConn1 -- Bus 1/RConn1
  Step-up Transformer 16.5 kV / 500 kV/RConn1 -- branch/LConn1
  Bus 2/LConn1 -- shunt/LConn1 -- Synchronous Machine GENTPJ Phasor/RConn1
  Bus 2/LConn2 -- shunt/LConn2 -- Synchronous Machine GENTPJ Phasor/RConn2
  Bus 2/LConn3 -- shunt/LConn3 -- Synchronous Machine GENTPJ Phasor/RConn3
  Bus 2/RConn1 -- Step-up Transformer 16.5 kV / 500 kV/LConn1
  Bus 2/RConn2 -- Step-up Transformer 16.5 kV / 500 kV/LConn2
  Bus 2/RConn3 -- Step-up Transformer 16.5 kV / 500 kV/LConn3

== system templateVFreplay/VF Replay/GOV/GGOV1 ==
  Pref : Inport
  meas : Inport  Port=2
  Bus Selector10 : BusSelector  OutputSignals="Mechanical.Rotor speed  wm  (pu),Mechanical.Electrical power  Pe (pu)"
  Gain1 : Gain  Gain=g.MBASE/p.mwcap
  Gain2 : Gain  Gain=p.mwcap/g.MBASE
  "General Governor (Continuous) " : Subsystem  mask(GGOV1 Governor Model){Tpelec=p.tpelec, Kpgov=p.kpgov, Kigov=p.kigov, Kdgov=p.kdgov, Tdgov=p.tdgov, errvec=[p.minerr p.maxerr], vvec=[p.vmin p.vmax], r=p.r, rselect=Electrical Power, Tact=p.tact, Kturb=p.kturb, wfnl=p.wfnl, Tb=p.tb, Tc=p.tc, Teng=p.teng, Flag=Fuel Flow Proportional to Speed, Tfload=p.tfload, Kpload=p.kpload, Kiload=p.kiload, Ldref=p.ldref, Dm=p.dm, rvec=[p.rclose p.ropen], Kimw=p.kimw, Pmwset=p.pmwset, aset=p.aset, Ka=p.ka, Ta=p.ta, db=p.db, Tsa=p.tsa, Tsb=p.tsb, rlimitvec=[p.rdown p.rup], Tau=1e-4}
      mask prompts: Tpelec "Tpelec, Electrical Power Transducer Time Constant [s]"; Kpgov "Kpgov, Proportional Gain"; Kigov "Kigov, Integral Gain"; Kdgov "Kdgov, Derivative Gain"; Tdgov "Tdgov, Derivative Time Constant [s]"; errvec "[minerr maxerr], Speed Error Limits"; vvec "[vmin vmax], Valve Limits"; r "r, Permanent droop [pu]"; rselect "Feedback for Droop"; Tact "Tact, Actuator Time Constant"; Kturb "Kturb, Turbine Gain"; wfnl "wfnl, No Load Fuel Flow [pu]"; Tb "Tb, Lag Time Constant [s]"; Tc "Tc, Lead Time Constant [s]"; Teng "Teng, Transport Lag for Diesel [s]"; Flag "Fuel Source Characteristic"; Tfload "Tfload, Time Constant [s]"; Kpload "Kpload, Proportional Gain"; Kiload "Kiload, Integral Gain"; Ldref "Ldref, Load Limiter Reference Value [pu]"; Dm "Dm, Speed Sensitivity Coefficient [pu]"; rvec "[rclose ropen], Valve Opening Rates [pu/s]"; Kimw "Kimw, Power Controller Gain"; Pmwset "Pmwset, Power Controller Setpoint [MW]"; aset "aset, Acceleration Limiter Setpoint [pu/s]"; Ka "Ka, Acceleration Limiter Gain"; Ta "Ta, Acceleration Limiter Time Constant [s]"; db "db, Speed Governor Dead Band"; Tsa "Tsa, Temperature Detection Lead [s]"; Tsb "Tsb, Temperature Detection Lag [s]"; rlimitvec "[rdown rup], Load Limit Rates"; Tau "Algebraic Loop Time Constant [s]"
      mask init:
      | minerr = errvec(1);   maxerr = errvec(2);
      | vmin = vvec(1);       vmax = vvec(2);
      | ropen = rvec(2);      rclose = rvec(1);
      | rdown = rlimitvec(1); rup = rlimitvec(2);
      mask TypeOptions rselect: Electrical Power | None - Isochronous Governor | Fuel Valve Stroke - True Stroke | Governor Ouput - Requested Stroke
      mask TypeOptions Flag: Fuel Flow Independent of Speed | Fuel Flow Proportional to Speed
      mask DialogControl Container9 Prompt: Governor
      mask DialogControl Container11 Prompt: Droop
      mask DialogControl Container12 Prompt: Turbine
      mask DialogControl Container13 Prompt: Load Limiter
      mask DialogControl Container16 Prompt: Additional Limits
      mask DialogControl Container8 Prompt: Other
      mask Display:
      | port_label('input',1,'Pref');
      | port_label('input',2,'Speed');
      | port_label('input',3,'Pe');
      | port_label('output',1,'Pmech');
      | 
      | color('blue');disp('GGOV1')
  Pm : Outport  VectorParamsAs1DForOutWhenUnconnected=off
  wires:
  Bus Selector10/1 -> "General Governor (Continuous) "/2(Speed)  "<Rotor speed  wm  (pu)>"
  Bus Selector10/2 -> Gain1/1  "<Electrical power  Pe (pu)>"
  Pref/1 -> "General Governor (Continuous) "/1(Pref)
  meas/1 -> Bus Selector10/1
  "General Governor (Continuous) "/1(Pmech) -> Gain2/1
  Gain1/1 -> "General Governor (Continuous) "/3(Pe)
  Gain2/1 -> Pm/1
